simulink model "ModelosTFG"  (R2024b)
settings: Solver=VariableStepAuto  StartTime=0.0  StopTime=75000  RelTol=1e-3
undefined symbols (not defined in the file): Gb, Ib, n, p1, p2, p3, Vi
libraries: slpidlib x2
settings Model: Creator=HP  LastModifiedBy=HP

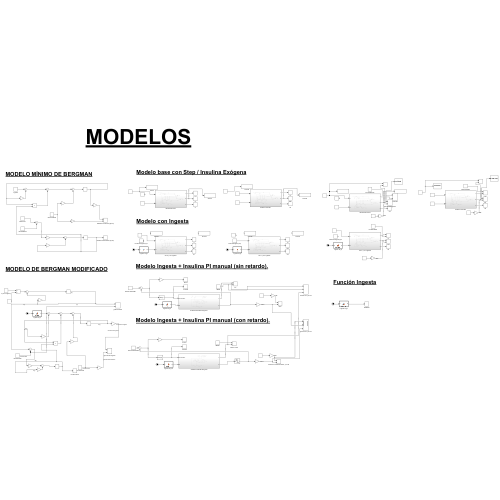
[thumbnail: Simulink's stored preview of the top-level diagram]
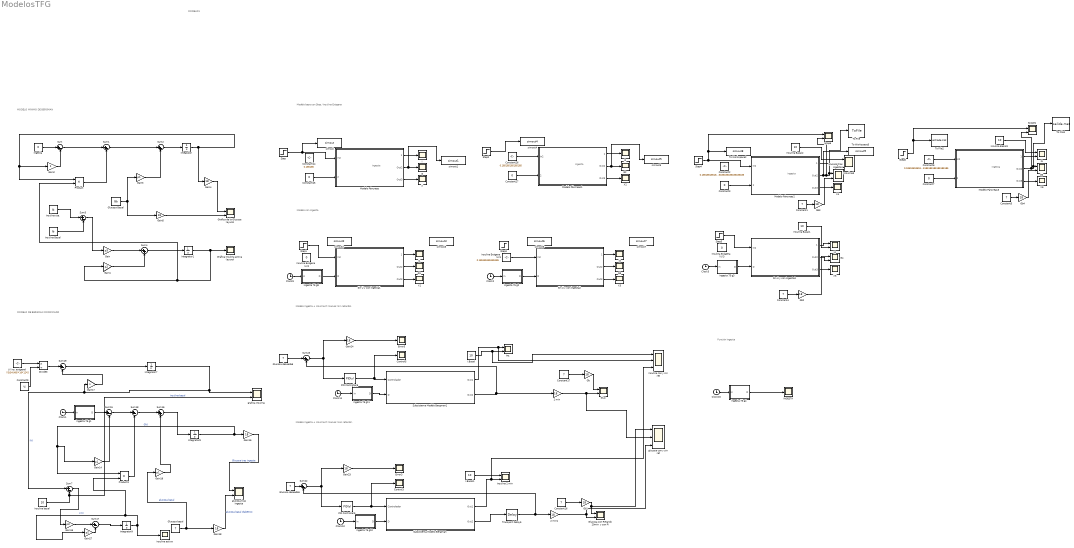
== system ModelosTFG ==
  note: ingesta
  note: Modelo Ingesta + Insulina PI manual (sin retardo).
  note: MODELOS
  note: Función Ingesta
  note: Modelo con Ingesta
  note: ingesta
  note: Modelo base con Step / Insulina Exógena
  note: Modelo Ingesta + Insulina PI manual (con retardo).
  note: MODELO MÍNIMO DE BERGMAN
  note: MODELO DE BERGMAN MODIFICADO
  note: ingesta
  note: ingesta
  2 min : Gain  Gain=18
  2 min1 : Gain  Gain=18
  Clock{1..3,9..11,15} (7 alike) : Clock
  Constant{1,4..5,16..17} (5 alike) : Constant  Value=7
  Constant14 : Constant  Value=0.185185
  Constant{3,7,15,27} (4 alike) : Constant  Value=0
  Constant2 : Constant  Value=0.185185185185185185185185185185
  Constant26 : Constant  Value=0.185185185185185
  Constant6 : Constant  Value=0.185185185185185185185185185185
  Constant9 : Constant  Value=Vi
  Control3 : Scope
  Control5 : Scope
  Divide3 : Product  Inputs=*/
  Error3 : Scope
  Error5 : Scope
  G{,1..3} (4 alike) : Scope
  G4 : Scope  NumInputPorts=2
  G5 : Scope  NumInputPorts=2
  Gain : Gain  Gain=p3
  Gain1 : Gain  Gain=p2
  Gain14 : Gain  Gain=p1
  Gain15 : Gain  Gain=p3
  Gain{4..5,16,18,23..24} (6 alike) : Gain  Gain=18
  Gain17 : Gain  Gain=n
  Gain19 : Gain  Gain=p1
  Gain2 : Gain
  Gain27 : Gain  Gain=p2
  Gain3 : Gain  Gain=p1
  Gb{,1..4} (5 alike) : Gain  Gain=18
  Gluc : Scope  NumInputPorts=2
  Glucosa Basal : Constant  Value=Gb
  Glucosa basal : Constant  Value=7
  Glucosa con Retardo 20min  y con PI : Scope  NumInputPorts=2
  Glucosa deseada5 : Constant  Value=7
  Glucosa deseada6 : Constant  Value=7
  Gráfica Insulina activa (ayuno) : Scope
  Gráfica de la Glucosa (ayuno) : Scope  NumInputPorts=2
  I{,1..3} (4 alike) : Scope
  I.Basal : Constant  Value=10
  I.Basal1 : Constant  Value=10
  I4 : Scope  NumInputPorts=2
  I5 : Scope  NumInputPorts=2
  INGESTA : Scope
  Ingesta : Constant  Value=0
  Ingesta 75 g1 : MATLAB Function  TreatAsAtomicUnit=on
  Ingesta 75 g10 : MATLAB Function  TreatAsAtomicUnit=on
  Ingesta 75 g11 : MATLAB Function  TreatAsAtomicUnit=on
  Ingesta 75 g2 : MATLAB Function  TreatAsAtomicUnit=on
  Ingesta 75 g3 : MATLAB Function  TreatAsAtomicUnit=on
  Ingesta 75 g4 : MATLAB Function  TreatAsAtomicUnit=on
  Ingesta 75 g9 : MATLAB Function  TreatAsAtomicUnit=on
  Ins. : Scope  NumInputPorts=2
  Insulina 2 min : Scope  NumInputPorts=2
  Insulina Basal : Constant  Value=Ib
  Insulina Basal1 : Constant  Value=10
  Insulina Basal2 : Constant  Value=10
  Insulina Basal3 : Constant  Value=10
  Insulina Exógena (U)1 : Constant  Value=0.185185185185185
  Insulina Exógena (U)2 : Constant  Value=0
  Insulina Exógena (U)3 : Constant  Value=0
  Insulina basal : Constant  Value=10
  Insulina cte. : Constant  Value=Ib
  Integrator : Integrator  InitialCondition=4.5
  Integrator1 : Integrator
  Integrator7 : Integrator  InitialCondition=10
  Integrator8 : Integrator  InitialCondition=7
  Integrator9 : Integrator
  Modelo Páncreas : Subsystem
  Modelo Páncreas1 : Subsystem
  Modelo Páncreas2 : Subsystem
  Modelo Páncreas3 : Subsystem
  PID Controller5 : slpidlib/PID Controller  Controller=PID  Form=Parallel  TimeDomain=Continuous-time  UseExternalTs=off  SampleTime=-1  IntegratorMethod=Forward Euler  FilterMethod=Forward Euler  ControllerParametersSource=internal  P=-0.3195  I=-0.3195/2998.95  UseKiTs=off  D=0  UseExternalDerivativeSource=off  N=10  UseFilter=on  TunerSelectOption=Transfer Function Based (PID Tuner App)  InitialConditionSource=internal  InitialConditionForIntegrator=0  InitialConditionForFilter=0  DifferentiatorICPrevScaledInput=0  ExternalReset=none  TrackingMode=off  Kt=1  LimitOutput=off  SatLimitsSource=internal  UpperSaturationLimit=inf  LowerSaturationLimit=-inf  LinearizeAsGain=on  AntiWindupMode=none  Kb=1  LimitIntegrator=off  UpperIntegratorSaturationLimit=inf  LowerIntegratorSaturationLimit=-inf  POutMin=[]  POutMax=[]  IOutMin=[]  IOutMax=[]  DOutMin=[]  DOutMax=[]  NOutMin=[]  NOutMax=[]  SumOutMin=[]  SumOutMax=[]  SaturationOutMin=[]  SaturationOutMax=[]  PParamMin=[]  PParamMax=[]  IParamMin=[]  IParamMax=[]  DParamMin=[]  DParamMax=[]  NParamMin=[]  NParamMax=[]  KbParamMin=[]  KbParamMax=[]  KtParamMin=[]  KtParamMax=[]  KbOutMin=[]  KbOutMax=[]  KtOutMin=[]  KtOutMax=[]  IntegratorOutMin=[]  IntegratorOutMax=[]  FilterOutMin=[]  FilterOutMax=[]  SumI1OutMin=[]  SumI1OutMax=[]  SumI2OutMin=[]  SumI2OutMax=[]  SumI3OutMin=[]  SumI3OutMax=[]  SumI4OutMin=[]  SumI4OutMax=[]  SumDOutMin=[]  SumDOutMax=[]  DifferentiatorOutMin=[]  DifferentiatorOutMax=[]  FilterDiffOutCoefMin=[]  FilterDiffOutCoefMax=[]  ReciprocalOutMin=[]  ReciprocalOutMax=[]  SumDenOutMin=[]  SumDenOutMax=[]  SumNumOutMin=[]  SumNumOutMax=[]  DivideOutMin=[]  DivideOutMax=[]  UdiffTsProdOutMin=[]  UdiffTsProdOutMax=[]  NTsProdOutMin=[]  NTsProdOutMax=[]  UintegralTsProdOutMin=[]  UintegralTsProdOutMax=[]  UngainTsProdOutMin=[]  UngainTsProdOutMax=[]  ClampingZeroOutDataTypeStr=Inherit: Inherit via back propagation  ClampingZeroOutMin=[]  ClampingZeroOutMax=[]  FilterDenConstantOutDataTypeStr=Inherit: Inherit via back propagation  FilterDenConstantOutMin=[]  FilterDenConstantOutMax=[]  PCopyOutDataTypeStr=Inherit: Inherit via back propagation  PCopyOutMin=[]  PCopyOutMax=[]  NCopyOutDataTypeStr=Inherit: Inherit via back propagation  NCopyOutMin=[]  NCopyOutMax=[]  IntegratorContinuousStateAttributes=''  IntegratorStateMustResolveToSignalObject=off  IntegratorRTWStateStorageClass=Auto  FilterContinuousStateAttributes=''  FilterStateMustResolveToSignalObject=off  FilterRTWStateStorageClass=Auto  ParallelPVariant=InternalParameters  IdealPVariant=Disabled  IVariant=InternalParameters  DVariant=InternalParameters  IntegratorVariant=Continuous  SatVariant=Disabled  AWVariant=Passthrough  PCopyVariant=Disabled  TRVariant=Disabled  FdbkBlocksVariant=Forward  IdealPFdbkVariant=Disabled  SatFdbkVariant=Disabled  DerivativeFilterVariant=ContFilter  NVariant=InternalParameters  NCopyVariant=Disabled  FilterICVariant=InternalICsFilter  IntegratorICVariant=InternalICs  ExternalResetVariant=Disabled  TRSumVariant=Passthrough  SumFdbkVariant=Disabled  SumVariant=Sum_PID  TsampFilterVariant=InternalTs  TsampNgainVariant=Passthrough  TsampIntegralVariant=Disabled_SignalSpec  ExternalSaturationOutDataTypeStr=Inherit: Same as second input  DerivativeSourceVariant=ErrorSignal  PreIntVariant=InternalPreInt
  PID Controller6 : slpidlib/PID Controller  Controller=PID  Form=Parallel  TimeDomain=Continuous-time  UseExternalTs=off  SampleTime=-1  IntegratorMethod=Forward Euler  FilterMethod=Forward Euler  ControllerParametersSource=internal  P=-0.3195  I=-0.3195/2998.95  UseKiTs=off  D=0  UseExternalDerivativeSource=off  N=10  UseFilter=on  TunerSelectOption=Transfer Function Based (PID Tuner App)  InitialConditionSource=internal  InitialConditionForIntegrator=0  InitialConditionForFilter=0  DifferentiatorICPrevScaledInput=0  ExternalReset=none  TrackingMode=off  Kt=1  LimitOutput=off  SatLimitsSource=internal  UpperSaturationLimit=inf  LowerSaturationLimit=-inf  LinearizeAsGain=on  AntiWindupMode=none  Kb=1  LimitIntegrator=off  UpperIntegratorSaturationLimit=inf  LowerIntegratorSaturationLimit=-inf  POutMin=[]  POutMax=[]  IOutMin=[]  IOutMax=[]  DOutMin=[]  DOutMax=[]  NOutMin=[]  NOutMax=[]  SumOutMin=[]  SumOutMax=[]  SaturationOutMin=[]  SaturationOutMax=[]  PParamMin=[]  PParamMax=[]  IParamMin=[]  IParamMax=[]  DParamMin=[]  DParamMax=[]  NParamMin=[]  NParamMax=[]  KbParamMin=[]  KbParamMax=[]  KtParamMin=[]  KtParamMax=[]  KbOutMin=[]  KbOutMax=[]  KtOutMin=[]  KtOutMax=[]  IntegratorOutMin=[]  IntegratorOutMax=[]  FilterOutMin=[]  FilterOutMax=[]  SumI1OutMin=[]  SumI1OutMax=[]  SumI2OutMin=[]  SumI2OutMax=[]  SumI3OutMin=[]  SumI3OutMax=[]  SumI4OutMin=[]  SumI4OutMax=[]  SumDOutMin=[]  SumDOutMax=[]  DifferentiatorOutMin=[]  DifferentiatorOutMax=[]  FilterDiffOutCoefMin=[]  FilterDiffOutCoefMax=[]  ReciprocalOutMin=[]  ReciprocalOutMax=[]  SumDenOutMin=[]  SumDenOutMax=[]  SumNumOutMin=[]  SumNumOutMax=[]  DivideOutMin=[]  DivideOutMax=[]  UdiffTsProdOutMin=[]  UdiffTsProdOutMax=[]  NTsProdOutMin=[]  NTsProdOutMax=[]  UintegralTsProdOutMin=[]  UintegralTsProdOutMax=[]  UngainTsProdOutMin=[]  UngainTsProdOutMax=[]  ClampingZeroOutDataTypeStr=Inherit: Inherit via back propagation  ClampingZeroOutMin=[]  ClampingZeroOutMax=[]  FilterDenConstantOutDataTypeStr=Inherit: Inherit via back propagation  FilterDenConstantOutMin=[]  FilterDenConstantOutMax=[]  PCopyOutDataTypeStr=Inherit: Inherit via back propagation  PCopyOutMin=[]  PCopyOutMax=[]  NCopyOutDataTypeStr=Inherit: Inherit via back propagation  NCopyOutMin=[]  NCopyOutMax=[]  IntegratorContinuousStateAttributes=''  IntegratorStateMustResolveToSignalObject=off  IntegratorRTWStateStorageClass=Auto  FilterContinuousStateAttributes=''  FilterStateMustResolveToSignalObject=off  FilterRTWStateStorageClass=Auto  ParallelPVariant=InternalParameters  IdealPVariant=Disabled  IVariant=InternalParameters  DVariant=InternalParameters  IntegratorVariant=Continuous  SatVariant=Disabled  AWVariant=Passthrough  PCopyVariant=Disabled  TRVariant=Disabled  FdbkBlocksVariant=Forward  IdealPFdbkVariant=Disabled  SatFdbkVariant=Disabled  DerivativeFilterVariant=ContFilter  NVariant=InternalParameters  NCopyVariant=Disabled  FilterICVariant=InternalICsFilter  IntegratorICVariant=InternalICs  ExternalResetVariant=Disabled  TRSumVariant=Passthrough  SumFdbkVariant=Disabled  SumVariant=Sum_PID  TsampFilterVariant=InternalTs  TsampNgainVariant=Passthrough  TsampIntegralVariant=Disabled_SignalSpec  ExternalSaturationOutDataTypeStr=Inherit: Same as second input  DerivativeSourceVariant=ErrorSignal  PreIntVariant=InternalPreInt
  Product : Product
  Product3 : Product
  Scope : Scope  NumInputPorts=2
  Scope1 : Scope  NumInputPorts=2
  Sin U y con Ingesta1 : Subsystem
  Sin U y con Ingesta2 : Subsystem
  Sin U y con Ingesta3 : Subsystem
  Step{,1..3,5} (5 alike) : Step  Time=100  Before=0.185185  After=1.185185  SampleTime=0
  Step4 : Step  Time=2000  Before=0.185185185185  After=1.185185  SampleTime=0
  Step6 : Step  Time=2000  Before=0.185185  After=1.185185  SampleTime=0
  Subsistema Modelo Bergman : Subsystem
  Subsistema Modelo Bergman1 : Subsystem
  Sum{,1,3,7,15,17..19,22..23} (10 alike) : Sum  Inputs=|+-
  Sum16 : Sum  Inputs=|++
  Sum2 : Sum  Inputs=|++
  Sum4 : Sum  Inputs=|++
  To File : ToFile  SampleTime=100
  To File1 : ToFile  Filename=salida.mat  MatrixName=glucosa
  To File2 : ToFile  Filename=entrada.mat  MatrixName=Insulina
  To Workspace2 : ToWorkspace  VariableName=simout8  SaveFormat=Timeseries  SampleTime=-1
  To Workspace3 : ToWorkspace  VariableName=simout9  SaveFormat=Timeseries  SampleTime=-1
  Transport Delay5 : TransportDelay  DelayTime=900  InitialOutput=7
  "U (ins. exógena) " : Constant  Value=((5/54)/60)*10*12*5
  X{,1..6} (7 alike) : Scope
  glucosa con y sin ret : Scope  NumInputPorts=3
  glucosa tras ingesta : Scope  NumInputPorts=2
  glucosa tras ingesta1 : Scope  NumInputPorts=2
  grafica insulina : Scope  NumInputPorts=2
  insulina activa : Scope
  insulina con y sin ret : Scope  NumInputPorts=3
  insulina3 : Scope  NumInputPorts=2
  simout : ToWorkspace  VariableName=simout  SaveFormat=Timeseries  SampleTime=-1
  simout1 : ToWorkspace  VariableName=simout1  SaveFormat=Timeseries  SampleTime=-1
  simout2 : ToWorkspace  VariableName=simout2  SaveFormat=Timeseries  SampleTime=-1
  simout3 : ToWorkspace  VariableName=simout3  SaveFormat=Timeseries  SampleTime=-1
  simout4 : ToWorkspace  VariableName=simout4  SaveFormat=Timeseries  SampleTime=-1
  simout5 : ToWorkspace  VariableName=simout5  SaveFormat=Timeseries  SampleTime=-1
  simout6 : ToWorkspace  VariableName=simout6  SaveFormat=Timeseries  SampleTime=-1
  simout7 : ToWorkspace  VariableName=simout7  SaveFormat=Timeseries  SampleTime=-1
  wires:
  Clock10/1 -> Ingesta 75 g10/1(in)
  Modelo Páncreas1/2(Out2) -> simout5/1, G2/1
  Modelo Páncreas/2(Out2) -> simout1/1, G/1
  Step2/1 -> simout4/1
  PID Controller6/1 -> Control5/1, Subsistema Modelo Bergman1/1(Controlador)
  Modelo Páncreas/1(1) -> I/1
  I.Basal1/1 -> Insulina 2 min/1
  Constant16/1 -> Gb1/1
  I.Basal/1 -> insulina con y sin ret/1, Ins./2
  Constant17/1 -> Gb/1
  Sum23/1 -> PID Controller6/1, Gain24/1
  Step/1 -> simout/1, Modelo Páncreas/1(In2)
  Glucosa deseada5/1 -> Sum22/1
  Ingesta 75 g11/1(D) -> Subsistema Modelo Bergman1/2(D)
  2 min/1 -> glucosa con y sin ret/2, Gluc/2
  Step1/1 -> Sin U y con Ingesta1/1(In2)
  Clock11/1 -> Ingesta 75 g11/1(in)
  2 min1/1 -> glucosa con y sin ret/3, Glucosa con Retardo 20min  y con PI/2
  Clock9/1 -> Ingesta 75 g9/1(in)
  Constant26/1 -> Modelo Páncreas1/1(In2)
  Ingesta 75 g9/1(D) -> Sin U y con Ingesta1/2(D)
  Gb1/1 -> Glucosa con Retardo 20min  y con PI/1, glucosa con y sin ret/1
  Sin U y con Ingesta1/1(1) -> I1/1
  Subsistema Modelo Bergman1/1(Out1) -> insulina con y sin ret/2, Ins./1
  Constant27/1 -> Modelo Páncreas1/2(2)
  Sin U y con Ingesta1/3(Out3) -> X1/1
  Sum22/1 -> PID Controller5/1, Gain23/1
  Glucosa deseada6/1 -> Sum23/1
  Gb/1 -> Gluc/1
  Subsistema Modelo Bergman1/2(Out2) -> Sum23/2, 2 min/1
  Modelo Páncreas1/1(1) -> I2/1
  Clock15/1 -> Ingesta 75 g4/1(in)
  PID Controller5/1 -> Control3/1, Subsistema Modelo Bergman/1(Controlador)
  Subsistema Modelo Bergman/2(Out2) -> Transport Delay5/1
  Modelo Páncreas/3(Out3) -> X/1
  Ingesta 75 g4/1(D) -> INGESTA/1
  Subsistema Modelo Bergman/1(Out1) -> insulina con y sin ret/3, Insulina 2 min/2
  Gain23/1 -> Error3/1
  Transport Delay5/1 -> Sum22/2, 2 min1/1
  Ingesta 75 g10/1(D) -> Subsistema Modelo Bergman/2(D)
  Modelo Páncreas1/3(Out3) -> X2/1
  Gain24/1 -> Error5/1
  Constant15/1 -> Modelo Páncreas/2(2)
  Sin U y con Ingesta1/2(Out2) -> G1/1
  Glucosa Basal/1 -> Gain3/1, Gain5/1
  Sum/1 -> Sum1/1
  Insulina cte./1 -> Sum3/1
  Sum4/1 -> Integrator1/1
  Ingesta/1 -> Sum/1
  Gain4/1 -> Gráfica de la Glucosa (ayuno)/1
  Sum2/1 -> Integrator/1
  Gain3/1 -> Sum2/2
  Gain1/1 -> Sum4/2
  Integrator/1 -> Gain4/1, Product/1, Gain2/1
  Sum3/1 -> Gain/1
  Gain/1 -> Sum4/1
  Integrator1/1 -> Product/2, Gain1/1, Gráfica Insulina activa (ayuno)/1
  Insulina Basal/1 -> Sum3/2
  Product/1 -> Sum1/2
  Sum1/1 -> Sum2/1
  Gain2/1 -> Sum/2
  Sum15/1 -> Sum18/1
  Integrator9/1 -> insulina activa/1, Product3/2, Gain27/1  "X(t)"
  Divide3/1 -> Sum19/1
  Gain14/1 -> Sum15/2
  Insulina basal/1 -> grafica insulina/2, Sum7/2  "insulina basal"
  Sum18/1 -> Sum16/1
  Gain27/1 -> Sum17/2
  Gain19/1 -> Sum16/2
  Glucosa basal/1 -> Gain19/1, Gain18/1  "glucosa basal"
  Integrator7/1 -> Sum7/1, Gain17/1, grafica insulina/1  "I(t)"
  Sum16/1 -> Integrator8/1
  Clock1/1 -> Ingesta 75 g1/1(in)
  Ingesta 75 g1/1(D) -> Sum15/1
  Integrator8/1 -> Gain16/1, Product3/1, Gain14/1  "G(t)"
  Gain17/1 -> Sum19/2
  Gain16/1 -> glucosa tras ingesta/1  "Glucosa tras ingesta"
  Product3/1 -> Sum18/2
  Gain18/1 -> glucosa tras ingesta/2  "glucosa basal diabetico"
  Sum17/1 -> Integrator9/1
  Sum19/1 -> Integrator7/1
  Sum7/1 -> Gain15/1
  "U (ins. exógena) "/1 -> Divide3/1
  Constant9/1 -> Divide3/2
  Gain15/1 -> Sum17/1
  Gain5/1 -> Gráfica de la Glucosa (ayuno)/2
  Sin U y con Ingesta2/2(Out2) -> G3/1
  Ingesta 75 g2/1(D) -> Sin U y con Ingesta2/2(D)
  Sin U y con Ingesta2/1(1) -> I3/1
  Sin U y con Ingesta2/3(Out3) -> X3/1
  Clock2/1 -> Ingesta 75 g2/1(in)
  Insulina Exógena (U)1/1 -> Sin U y con Ingesta2/1(In2)
  Insulina Basal2/1 -> insulina3/1
  Modelo Páncreas2/1(1) -> insulina3/2
  Gb3/1 -> glucosa tras ingesta1/2
  Modelo Páncreas2/2(Out2) -> To Workspace3/1, Scope/2, glucosa tras ingesta1/1, To File/1
  Step5/1 -> Sin U y con Ingesta3/1(In2)
  Modelo Páncreas3/2(Out2) -> Scope1/2, G5/1, To File1/1
  Modelo Páncreas3/3(Out3) -> X6/1
  Sin U y con Ingesta3/1(1) -> I4/1
  Constant3/1 -> Modelo Páncreas2/2(2)
  Modelo Páncreas3/1(1) -> I5/2
  Constant6/1 -> Modelo Páncreas3/1(In2)
  Step4/1 -> To Workspace2/1, Scope/1, Modelo Páncreas2/1(In2)
  Insulina Basal3/1 -> I5/1
  Sin U y con Ingesta3/2(Out2) -> G4/2
  Insulina Basal1/1 -> I4/2
  Gb4/1 -> G5/2
  Gb2/1 -> G4/1
  Ingesta 75 g3/1(D) -> Sin U y con Ingesta3/2(D)
  Constant5/1 -> Gb4/1
  Clock3/1 -> Ingesta 75 g3/1(in)
  Sin U y con Ingesta3/3(Out3) -> X5/1
  Step6/1 -> Scope1/1, To File2/1
  Constant7/1 -> Modelo Páncreas3/2(2)
  Constant1/1 -> Gb3/1
  Constant4/1 -> Gb2/1
  Modelo Páncreas2/3(Out3) -> X4/1

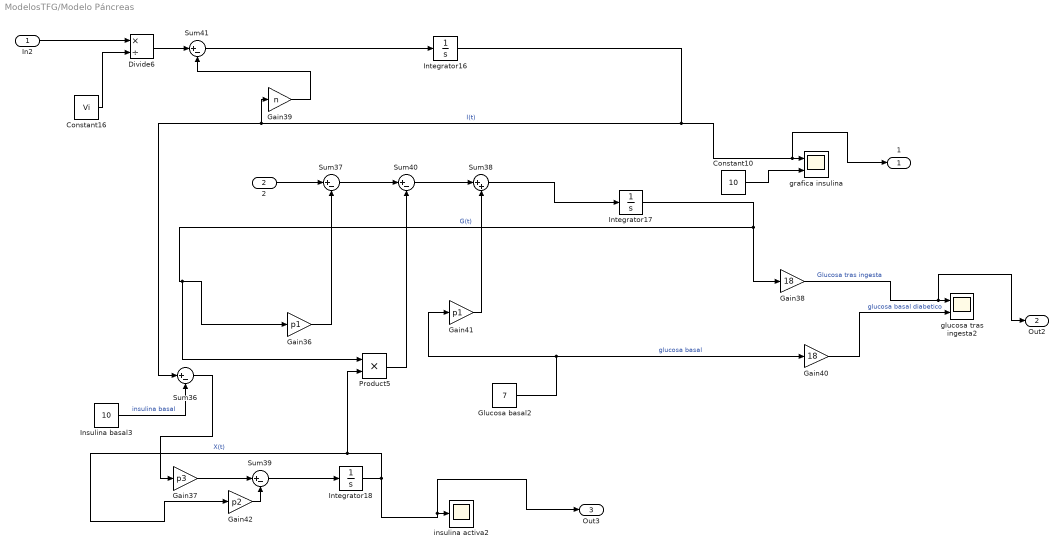
== system ModelosTFG/Modelo Páncreas ==
  In2 : Inport
  2 : Inport  Port=2
  Constant10 : Constant  Value=10
  Constant16 : Constant  Value=Vi
  Divide6 : Product  Inputs=*/
  Gain36 : Gain  Gain=p1
  Gain37 : Gain  Gain=p3
  Gain38 : Gain  Gain=18
  Gain39 : Gain  Gain=n
  Gain40 : Gain  Gain=18
  Gain41 : Gain  Gain=p1
  Gain42 : Gain  Gain=p2
  Glucosa basal2 : Constant  Value=7
  Insulina basal3 : Constant  Value=10
  Integrator16 : Integrator  InitialCondition=10
  Integrator17 : Integrator  InitialCondition=7
  Integrator18 : Integrator
  Product5 : Product
  Sum{36..37,39..41} (5 alike) : Sum  Inputs=|+-
  Sum38 : Sum  Inputs=|++
  glucosa tras ingesta2 : Scope  NumInputPorts=2
  grafica insulina : Scope  NumInputPorts=2
  insulina activa2 : Scope
  1 : Outport
  Out2 : Outport  Port=2
  Out3 : Outport  Port=3
  wires:
  Integrator18/1 -> Out3/1, insulina activa2/1, Product5/2, Gain42/1  "X(t)"
  Integrator17/1 -> Gain38/1, Product5/1, Gain36/1  "G(t)"
  Gain39/1 -> Sum41/2
  Glucosa basal2/1 -> Gain41/1, Gain40/1  "glucosa basal"
  Integrator16/1 -> Sum36/1, Gain39/1, 1/1, grafica insulina/1  "I(t)"
  Constant10/1 -> grafica insulina/2
  Gain42/1 -> Sum39/2
  2/1 -> Sum37/1
  Sum37/1 -> Sum40/1
  Sum39/1 -> Integrator18/1
  Gain40/1 -> glucosa tras ingesta2/2  "glucosa basal diabetico"
  Sum40/1 -> Sum38/1
  In2/1 -> Divide6/1
  Gain36/1 -> Sum37/2
  Gain38/1 -> Out2/1, glucosa tras ingesta2/1  "Glucosa tras ingesta"
  Sum36/1 -> Gain37/1
  Gain41/1 -> Sum38/2
  Gain37/1 -> Sum39/1
  Sum41/1 -> Integrator16/1
  Sum38/1 -> Integrator17/1
  Insulina basal3/1 -> Sum36/2  "insulina basal"
  Divide6/1 -> Sum41/1
  Constant16/1 -> Divide6/2
  Product5/1 -> Sum40/2

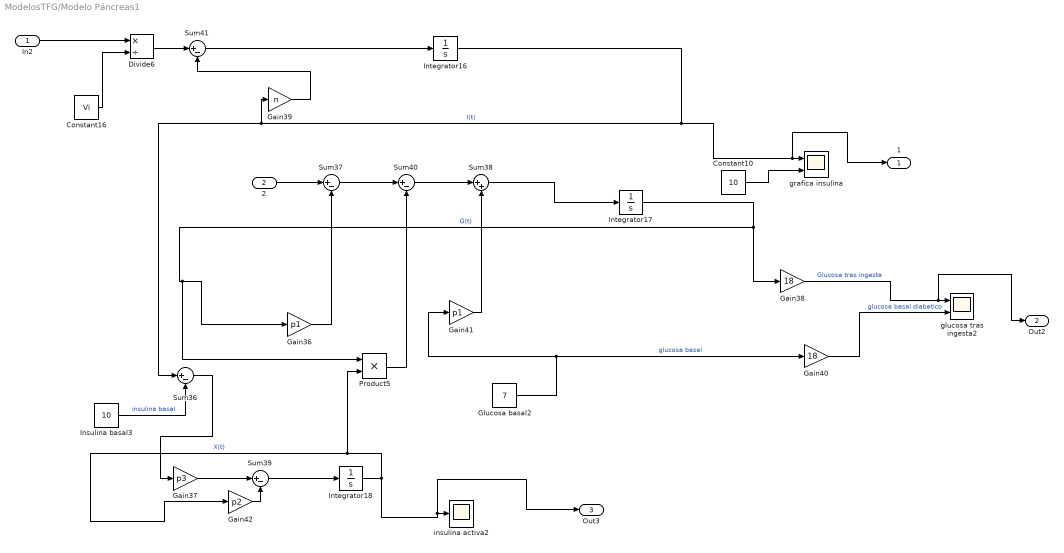
== system ModelosTFG/Modelo Páncreas1 ==
  In2 : Inport
  2 : Inport  Port=2
  Constant10 : Constant  Value=10
  Constant16 : Constant  Value=Vi
  Divide6 : Product  Inputs=*/
  Gain36 : Gain  Gain=p1
  Gain37 : Gain  Gain=p3
  Gain38 : Gain  Gain=18
  Gain39 : Gain  Gain=n
  Gain40 : Gain  Gain=18
  Gain41 : Gain  Gain=p1
  Gain42 : Gain  Gain=p2
  Glucosa basal2 : Constant  Value=7
  Insulina basal3 : Constant  Value=10
  Integrator16 : Integrator  InitialCondition=10
  Integrator17 : Integrator  InitialCondition=7
  Integrator18 : Integrator
  Product5 : Product
  Sum{36..37,39..41} (5 alike) : Sum  Inputs=|+-
  Sum38 : Sum  Inputs=|++
  glucosa tras ingesta2 : Scope  NumInputPorts=2
  grafica insulina : Scope  NumInputPorts=2
  insulina activa2 : Scope
  1 : Outport
  Out2 : Outport  Port=2
  Out3 : Outport  Port=3
  wires:
  Integrator18/1 -> Out3/1, insulina activa2/1, Product5/2, Gain42/1  "X(t)"
  Integrator17/1 -> Gain38/1, Product5/1, Gain36/1  "G(t)"
  Gain39/1 -> Sum41/2
  Glucosa basal2/1 -> Gain41/1, Gain40/1  "glucosa basal"
  Integrator16/1 -> Sum36/1, Gain39/1, 1/1, grafica insulina/1  "I(t)"
  Constant10/1 -> grafica insulina/2
  Gain42/1 -> Sum39/2
  2/1 -> Sum37/1
  Sum37/1 -> Sum40/1
  Sum39/1 -> Integrator18/1
  Gain40/1 -> glucosa tras ingesta2/2  "glucosa basal diabetico"
  Sum40/1 -> Sum38/1
  In2/1 -> Divide6/1
  Gain36/1 -> Sum37/2
  Gain38/1 -> Out2/1, glucosa tras ingesta2/1  "Glucosa tras ingesta"
  Sum36/1 -> Gain37/1
  Gain41/1 -> Sum38/2
  Gain37/1 -> Sum39/1
  Sum41/1 -> Integrator16/1
  Sum38/1 -> Integrator17/1
  Insulina basal3/1 -> Sum36/2  "insulina basal"
  Divide6/1 -> Sum41/1
  Constant16/1 -> Divide6/2
  Product5/1 -> Sum40/2

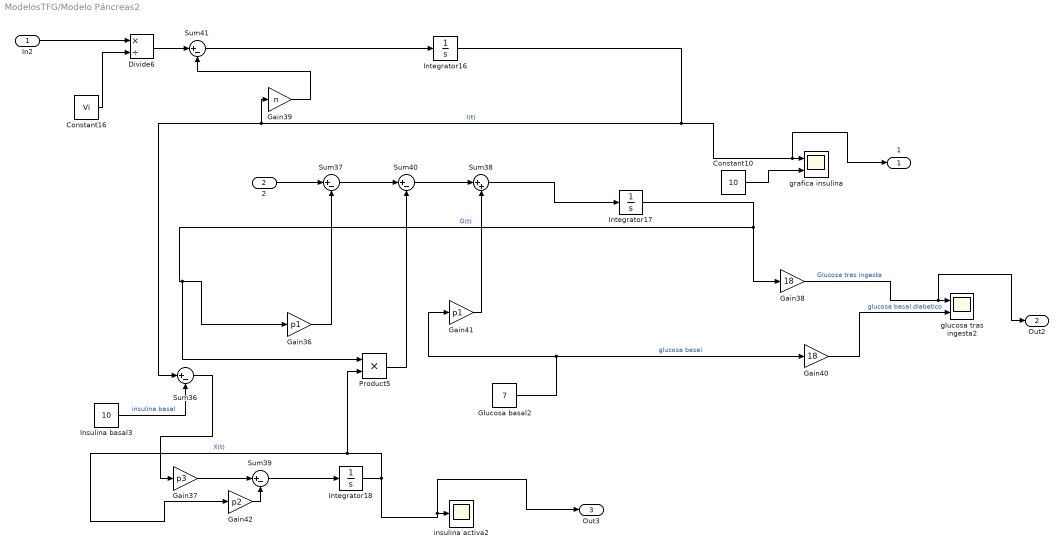
== system ModelosTFG/Modelo Páncreas2 ==
  In2 : Inport
  2 : Inport  Port=2
  Constant10 : Constant  Value=10
  Constant16 : Constant  Value=Vi
  Divide6 : Product  Inputs=*/
  Gain36 : Gain  Gain=p1
  Gain37 : Gain  Gain=p3
  Gain38 : Gain  Gain=18
  Gain39 : Gain  Gain=n
  Gain40 : Gain  Gain=18
  Gain41 : Gain  Gain=p1
  Gain42 : Gain  Gain=p2
  Glucosa basal2 : Constant  Value=7
  Insulina basal3 : Constant  Value=10
  Integrator16 : Integrator  InitialCondition=10
  Integrator17 : Integrator  InitialCondition=7
  Integrator18 : Integrator
  Product5 : Product
  Sum{36..37,39..41} (5 alike) : Sum  Inputs=|+-
  Sum38 : Sum  Inputs=|++
  glucosa tras ingesta2 : Scope  NumInputPorts=2
  grafica insulina : Scope  NumInputPorts=2
  insulina activa2 : Scope
  1 : Outport
  Out2 : Outport  Port=2
  Out3 : Outport  Port=3
  wires:
  Integrator18/1 -> Out3/1, insulina activa2/1, Product5/2, Gain42/1  "X(t)"
  Integrator17/1 -> Gain38/1, Product5/1, Gain36/1  "G(t)"
  Gain39/1 -> Sum41/2
  Glucosa basal2/1 -> Gain41/1, Gain40/1  "glucosa basal"
  Integrator16/1 -> Sum36/1, Gain39/1, 1/1, grafica insulina/1  "I(t)"
  Constant10/1 -> grafica insulina/2
  Gain42/1 -> Sum39/2
  2/1 -> Sum37/1
  Sum37/1 -> Sum40/1
  Sum39/1 -> Integrator18/1
  Gain40/1 -> glucosa tras ingesta2/2  "glucosa basal diabetico"
  Sum40/1 -> Sum38/1
  In2/1 -> Divide6/1
  Gain36/1 -> Sum37/2
  Gain38/1 -> Out2/1, glucosa tras ingesta2/1  "Glucosa tras ingesta"
  Sum36/1 -> Gain37/1
  Gain41/1 -> Sum38/2
  Gain37/1 -> Sum39/1
  Sum41/1 -> Integrator16/1
  Sum38/1 -> Integrator17/1
  Insulina basal3/1 -> Sum36/2  "insulina basal"
  Divide6/1 -> Sum41/1
  Constant16/1 -> Divide6/2
  Product5/1 -> Sum40/2

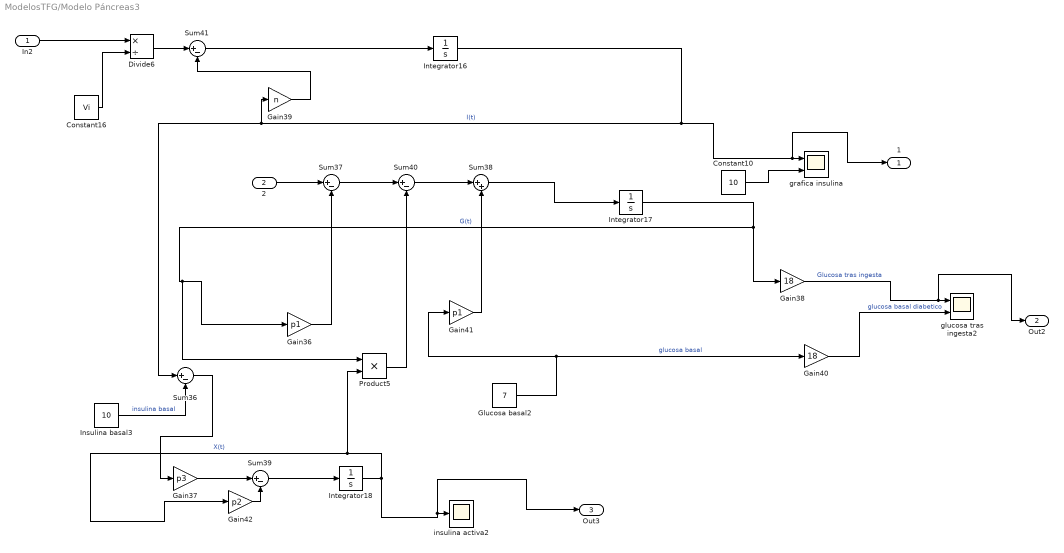
== system ModelosTFG/Modelo Páncreas3 ==
  In2 : Inport
  2 : Inport  Port=2
  Constant10 : Constant  Value=10
  Constant16 : Constant  Value=Vi
  Divide6 : Product  Inputs=*/
  Gain36 : Gain  Gain=p1
  Gain37 : Gain  Gain=p3
  Gain38 : Gain  Gain=18
  Gain39 : Gain  Gain=n
  Gain40 : Gain  Gain=18
  Gain41 : Gain  Gain=p1
  Gain42 : Gain  Gain=p2
  Glucosa basal2 : Constant  Value=7
  Insulina basal3 : Constant  Value=10
  Integrator16 : Integrator  InitialCondition=10
  Integrator17 : Integrator  InitialCondition=7
  Integrator18 : Integrator
  Product5 : Product
  Sum{36..37,39..41} (5 alike) : Sum  Inputs=|+-
  Sum38 : Sum  Inputs=|++
  glucosa tras ingesta2 : Scope  NumInputPorts=2
  grafica insulina : Scope  NumInputPorts=2
  insulina activa2 : Scope
  1 : Outport
  Out2 : Outport  Port=2
  Out3 : Outport  Port=3
  wires:
  Integrator18/1 -> Out3/1, insulina activa2/1, Product5/2, Gain42/1  "X(t)"
  Integrator17/1 -> Gain38/1, Product5/1, Gain36/1  "G(t)"
  Gain39/1 -> Sum41/2
  Glucosa basal2/1 -> Gain41/1, Gain40/1  "glucosa basal"
  Integrator16/1 -> Sum36/1, Gain39/1, 1/1, grafica insulina/1  "I(t)"
  Constant10/1 -> grafica insulina/2
  Gain42/1 -> Sum39/2
  2/1 -> Sum37/1
  Sum37/1 -> Sum40/1
  Sum39/1 -> Integrator18/1
  Gain40/1 -> glucosa tras ingesta2/2  "glucosa basal diabetico"
  Sum40/1 -> Sum38/1
  In2/1 -> Divide6/1
  Gain36/1 -> Sum37/2
  Gain38/1 -> Out2/1, glucosa tras ingesta2/1  "Glucosa tras ingesta"
  Sum36/1 -> Gain37/1
  Gain41/1 -> Sum38/2
  Gain37/1 -> Sum39/1
  Sum41/1 -> Integrator16/1
  Sum38/1 -> Integrator17/1
  Insulina basal3/1 -> Sum36/2  "insulina basal"
  Divide6/1 -> Sum41/1
  Constant16/1 -> Divide6/2
  Product5/1 -> Sum40/2

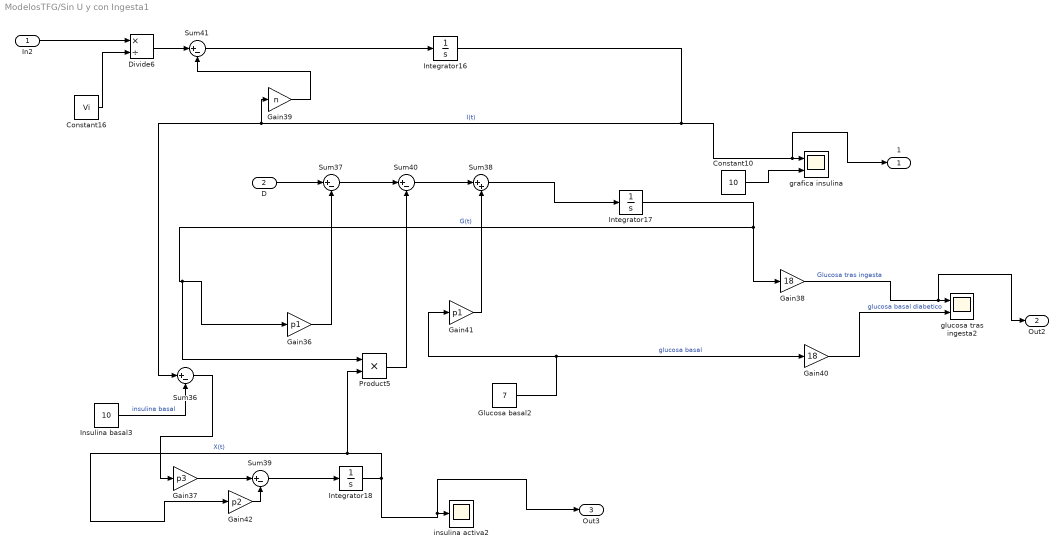
== system ModelosTFG/Sin U y con Ingesta1 ==
  In2 : Inport
  D : Inport  Port=2
  Constant10 : Constant  Value=10
  Constant16 : Constant  Value=Vi
  Divide6 : Product  Inputs=*/
  Gain36 : Gain  Gain=p1
  Gain37 : Gain  Gain=p3
  Gain38 : Gain  Gain=18
  Gain39 : Gain  Gain=n
  Gain40 : Gain  Gain=18
  Gain41 : Gain  Gain=p1
  Gain42 : Gain  Gain=p2
  Glucosa basal2 : Constant  Value=7
  Insulina basal3 : Constant  Value=10
  Integrator16 : Integrator  InitialCondition=10
  Integrator17 : Integrator  InitialCondition=7
  Integrator18 : Integrator
  Product5 : Product
  Sum{36..37,39..41} (5 alike) : Sum  Inputs=|+-
  Sum38 : Sum  Inputs=|++
  glucosa tras ingesta2 : Scope  NumInputPorts=2
  grafica insulina : Scope  NumInputPorts=2
  insulina activa2 : Scope
  1 : Outport
  Out2 : Outport  Port=2
  Out3 : Outport  Port=3
  wires:
  Integrator18/1 -> Out3/1, insulina activa2/1, Product5/2, Gain42/1  "X(t)"
  Integrator17/1 -> Gain38/1, Product5/1, Gain36/1  "G(t)"
  Gain39/1 -> Sum41/2
  Glucosa basal2/1 -> Gain41/1, Gain40/1  "glucosa basal"
  Integrator16/1 -> Sum36/1, Gain39/1, 1/1, grafica insulina/1  "I(t)"
  Constant10/1 -> grafica insulina/2
  Gain42/1 -> Sum39/2
  D/1 -> Sum37/1
  Sum37/1 -> Sum40/1
  Sum39/1 -> Integrator18/1
  Gain40/1 -> glucosa tras ingesta2/2  "glucosa basal diabetico"
  Sum40/1 -> Sum38/1
  In2/1 -> Divide6/1
  Gain36/1 -> Sum37/2
  Gain38/1 -> Out2/1, glucosa tras ingesta2/1  "Glucosa tras ingesta"
  Sum36/1 -> Gain37/1
  Gain41/1 -> Sum38/2
  Gain37/1 -> Sum39/1
  Sum41/1 -> Integrator16/1
  Sum38/1 -> Integrator17/1
  Insulina basal3/1 -> Sum36/2  "insulina basal"
  Divide6/1 -> Sum41/1
  Constant16/1 -> Divide6/2
  Product5/1 -> Sum40/2

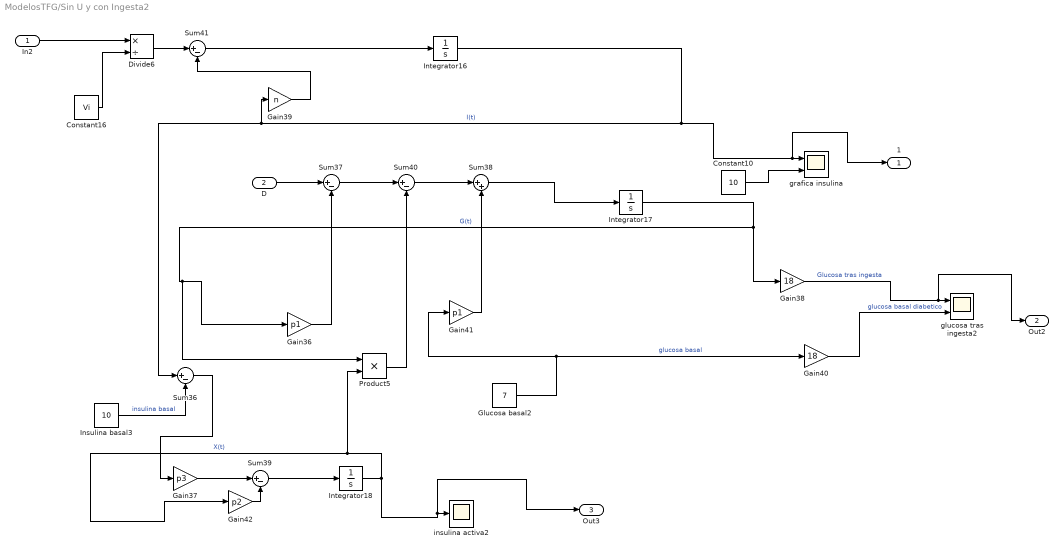
== system ModelosTFG/Sin U y con Ingesta2 ==
  In2 : Inport
  D : Inport  Port=2
  Constant10 : Constant  Value=10
  Constant16 : Constant  Value=Vi
  Divide6 : Product  Inputs=*/
  Gain36 : Gain  Gain=p1
  Gain37 : Gain  Gain=p3
  Gain38 : Gain  Gain=18
  Gain39 : Gain  Gain=n
  Gain40 : Gain  Gain=18
  Gain41 : Gain  Gain=p1
  Gain42 : Gain  Gain=p2
  Glucosa basal2 : Constant  Value=7
  Insulina basal3 : Constant  Value=10
  Integrator16 : Integrator  InitialCondition=10
  Integrator17 : Integrator  InitialCondition=7
  Integrator18 : Integrator
  Product5 : Product
  Sum{36..37,39..41} (5 alike) : Sum  Inputs=|+-
  Sum38 : Sum  Inputs=|++
  glucosa tras ingesta2 : Scope  NumInputPorts=2
  grafica insulina : Scope  NumInputPorts=2
  insulina activa2 : Scope
  1 : Outport
  Out2 : Outport  Port=2
  Out3 : Outport  Port=3
  wires:
  Integrator18/1 -> Out3/1, insulina activa2/1, Product5/2, Gain42/1  "X(t)"
  Integrator17/1 -> Gain38/1, Product5/1, Gain36/1  "G(t)"
  Gain39/1 -> Sum41/2
  Glucosa basal2/1 -> Gain41/1, Gain40/1  "glucosa basal"
  Integrator16/1 -> Sum36/1, Gain39/1, 1/1, grafica insulina/1  "I(t)"
  Constant10/1 -> grafica insulina/2
  Gain42/1 -> Sum39/2
  D/1 -> Sum37/1
  Sum37/1 -> Sum40/1
  Sum39/1 -> Integrator18/1
  Gain40/1 -> glucosa tras ingesta2/2  "glucosa basal diabetico"
  Sum40/1 -> Sum38/1
  In2/1 -> Divide6/1
  Gain36/1 -> Sum37/2
  Gain38/1 -> Out2/1, glucosa tras ingesta2/1  "Glucosa tras ingesta"
  Sum36/1 -> Gain37/1
  Gain41/1 -> Sum38/2
  Gain37/1 -> Sum39/1
  Sum41/1 -> Integrator16/1
  Sum38/1 -> Integrator17/1
  Insulina basal3/1 -> Sum36/2  "insulina basal"
  Divide6/1 -> Sum41/1
  Constant16/1 -> Divide6/2
  Product5/1 -> Sum40/2

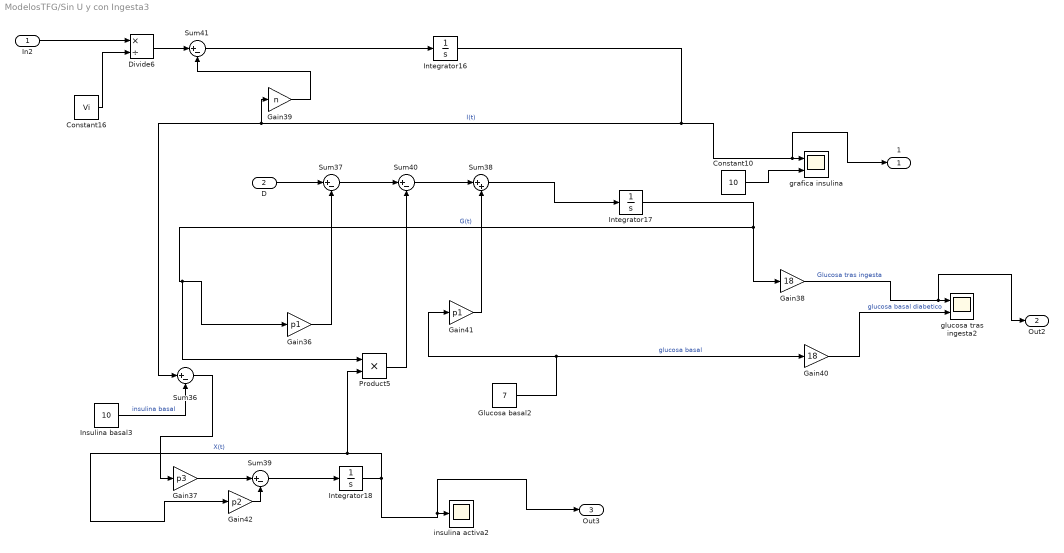
== system ModelosTFG/Sin U y con Ingesta3 ==
  In2 : Inport
  D : Inport  Port=2
  Constant10 : Constant  Value=10
  Constant16 : Constant  Value=Vi
  Divide6 : Product  Inputs=*/
  Gain36 : Gain  Gain=p1
  Gain37 : Gain  Gain=p3
  Gain38 : Gain  Gain=18
  Gain39 : Gain  Gain=n
  Gain40 : Gain  Gain=18
  Gain41 : Gain  Gain=p1
  Gain42 : Gain  Gain=p2
  Glucosa basal2 : Constant  Value=7
  Insulina basal3 : Constant  Value=10
  Integrator16 : Integrator  InitialCondition=10
  Integrator17 : Integrator  InitialCondition=7
  Integrator18 : Integrator
  Product5 : Product
  Sum{36..37,39..41} (5 alike) : Sum  Inputs=|+-
  Sum38 : Sum  Inputs=|++
  glucosa tras ingesta2 : Scope  NumInputPorts=2
  grafica insulina : Scope  NumInputPorts=2
  insulina activa2 : Scope
  1 : Outport
  Out2 : Outport  Port=2
  Out3 : Outport  Port=3
  wires:
  Integrator18/1 -> Out3/1, insulina activa2/1, Product5/2, Gain42/1  "X(t)"
  Integrator17/1 -> Gain38/1, Product5/1, Gain36/1  "G(t)"
  Gain39/1 -> Sum41/2
  Glucosa basal2/1 -> Gain41/1, Gain40/1  "glucosa basal"
  Integrator16/1 -> Sum36/1, Gain39/1, 1/1, grafica insulina/1  "I(t)"
  Constant10/1 -> grafica insulina/2
  Gain42/1 -> Sum39/2
  D/1 -> Sum37/1
  Sum37/1 -> Sum40/1
  Sum39/1 -> Integrator18/1
  Gain40/1 -> glucosa tras ingesta2/2  "glucosa basal diabetico"
  Sum40/1 -> Sum38/1
  In2/1 -> Divide6/1
  Gain36/1 -> Sum37/2
  Gain38/1 -> Out2/1, glucosa tras ingesta2/1  "Glucosa tras ingesta"
  Sum36/1 -> Gain37/1
  Gain41/1 -> Sum38/2
  Gain37/1 -> Sum39/1
  Sum41/1 -> Integrator16/1
  Sum38/1 -> Integrator17/1
  Insulina basal3/1 -> Sum36/2  "insulina basal"
  Divide6/1 -> Sum41/1
  Constant16/1 -> Divide6/2
  Product5/1 -> Sum40/2

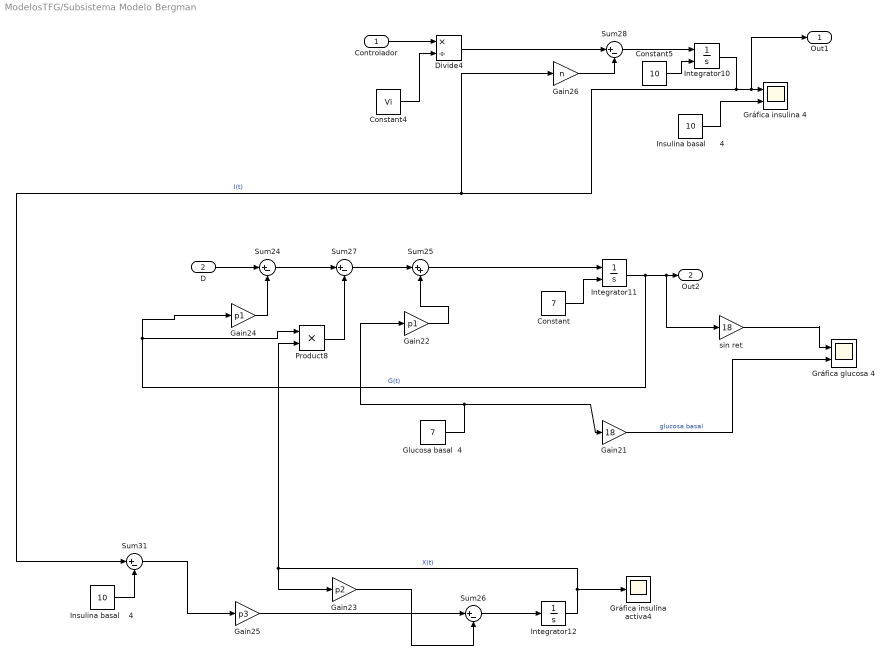
== system ModelosTFG/Subsistema Modelo Bergman ==
  Controlador : Inport
  D : Inport  Port=2
  Constant : Constant  Value=7
  Constant4 : Constant  Value=Vi
  Constant5 : Constant  Value=10
  Divide4 : Product  Inputs=*/
  Gain21 : Gain  Gain=18
  Gain22 : Gain  Gain=p1
  Gain23 : Gain  Gain=p2
  Gain24 : Gain  Gain=p1
  Gain25 : Gain  Gain=p3
  Gain26 : Gain  Gain=n
  Glucosa basal  4 : Constant  Value=7
  Gráfica glucosa 4 : Scope  NumInputPorts=2
  Gráfica insulina 4 : Scope  NumInputPorts=2
  Gráfica insulina activa4 : Scope
  Insulina basal      4 : Constant  Value=10
  Insulina basal    4 : Constant  Value=10
  Integrator10 : Integrator  InitialConditionSource=external
  Integrator11 : Integrator  InitialConditionSource=external  InitialCondition=7
  Integrator12 : Integrator
  Product8 : Product
  Sum{24,26..28,31} (5 alike) : Sum  Inputs=|+-
  Sum25 : Sum  Inputs=|++
  sin ret : Gain  Gain=18
  Out1 : Outport
  Out2 : Outport  Port=2
  wires:
  Gain26/1 -> Sum28/2
  Glucosa basal  4/1 -> Gain22/1, Gain21/1
  D/1 -> Sum24/1
  Gain21/1 -> Gráfica glucosa 4/2  "glucosa basal"
  Integrator11/1 -> sin ret/1, Out2/1, Gain24/1, Product8/1  "G(t)"
  Integrator12/1 -> Product8/2, Gain23/1, Gráfica insulina activa4/1  "X(t)"
  Gain25/1 -> Sum26/1
  Integrator10/1 -> Out1/1, Gráfica insulina 4/1, Sum31/1, Gain26/1  "I(t)"
  Constant5/1 -> Integrator10/2
  Sum31/1 -> Gain25/1
  Sum26/1 -> Integrator12/1
  Gain23/1 -> Sum26/2
  Sum28/1 -> Integrator10/1
  Sum24/1 -> Sum27/1
  Sum25/1 -> Integrator11/1
  Gain24/1 -> Sum24/2
  Insulina basal      4/1 -> Gráfica insulina 4/2
  Sum27/1 -> Sum25/1
  Insulina basal    4/1 -> Sum31/2
  Divide4/1 -> Sum28/1
  Gain22/1 -> Sum25/2
  Product8/1 -> Sum27/2
  Constant4/1 -> Divide4/2
  Constant/1 -> Integrator11/2
  Controlador/1 -> Divide4/1
  sin ret/1 -> Gráfica glucosa 4/1

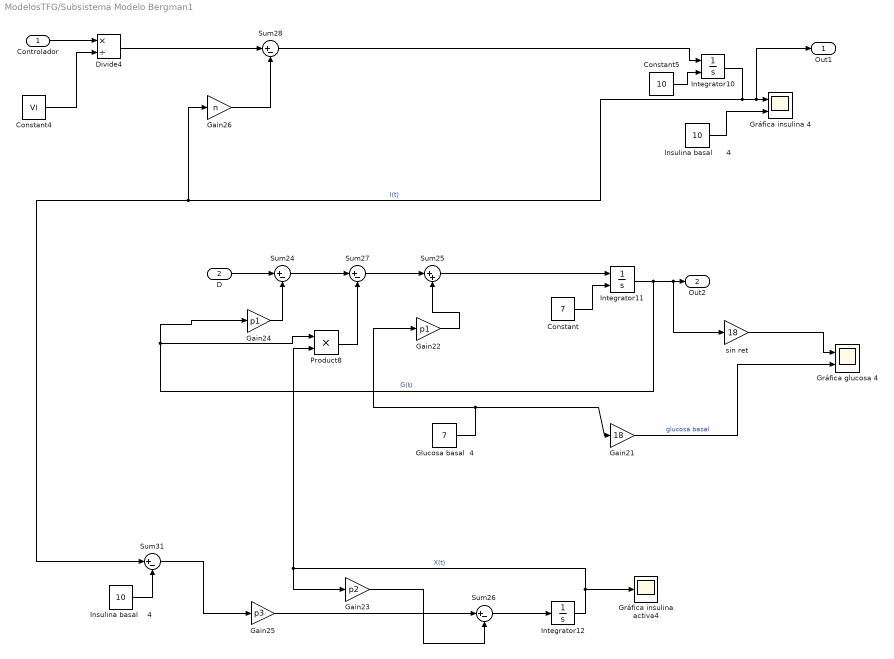
== system ModelosTFG/Subsistema Modelo Bergman1 ==
  Controlador : Inport
  D : Inport  Port=2
  Constant : Constant  Value=7
  Constant4 : Constant  Value=Vi
  Constant5 : Constant  Value=10
  Divide4 : Product  Inputs=*/
  Gain21 : Gain  Gain=18
  Gain22 : Gain  Gain=p1
  Gain23 : Gain  Gain=p2
  Gain24 : Gain  Gain=p1
  Gain25 : Gain  Gain=p3
  Gain26 : Gain  Gain=n
  Glucosa basal  4 : Constant  Value=7
  Gráfica glucosa 4 : Scope  NumInputPorts=2
  Gráfica insulina 4 : Scope  NumInputPorts=2
  Gráfica insulina activa4 : Scope
  Insulina basal      4 : Constant  Value=10
  Insulina basal    4 : Constant  Value=10
  Integrator10 : Integrator  InitialConditionSource=external
  Integrator11 : Integrator  InitialConditionSource=external  InitialCondition=7
  Integrator12 : Integrator
  Product8 : Product
  Sum{24,26..28,31} (5 alike) : Sum  Inputs=|+-
  Sum25 : Sum  Inputs=|++
  sin ret : Gain  Gain=18
  Out1 : Outport
  Out2 : Outport  Port=2
  wires:
  Gain26/1 -> Sum28/2
  Glucosa basal  4/1 -> Gain22/1, Gain21/1
  D/1 -> Sum24/1
  Gain21/1 -> Gráfica glucosa 4/2  "glucosa basal"
  Integrator11/1 -> sin ret/1, Out2/1, Gain24/1, Product8/1  "G(t)"
  Integrator12/1 -> Product8/2, Gain23/1, Gráfica insulina activa4/1  "X(t)"
  Gain25/1 -> Sum26/1
  Integrator10/1 -> Out1/1, Gráfica insulina 4/1, Sum31/1, Gain26/1  "I(t)"
  Constant5/1 -> Integrator10/2
  Sum31/1 -> Gain25/1
  Sum26/1 -> Integrator12/1
  Gain23/1 -> Sum26/2
  Sum28/1 -> Integrator10/1
  Sum24/1 -> Sum27/1
  Sum25/1 -> Integrator11/1
  Gain24/1 -> Sum24/2
  Insulina basal      4/1 -> Gráfica insulina 4/2
  Sum27/1 -> Sum25/1
  Insulina basal    4/1 -> Sum31/2
  Divide4/1 -> Sum28/1
  Gain22/1 -> Sum25/2
  Product8/1 -> Sum27/2
  Constant4/1 -> Divide4/2
  Constant/1 -> Integrator11/2
  Controlador/1 -> Divide4/1
  sin ret/1 -> Gráfica glucosa 4/1

== matlab function ModelosTFG/Ingesta 75 g2 ==
  data: in input; D output
function D = comida(in)
% Variables de entrada en la funcion
t = in(1) %- 8*60*60; % Ajuste para iniciar a las 8 de la mañana
 
% Parámetros del modelo
Ag = 0.8; % adimensional
Tmaxi = 55*60; % s
Vg = 13.79; % L
Tmaxg = 40*60; % s
t1 = 0;
Dg = 0;
f = 1000/180; % factor de conversión de g a mmol
 
% Comidas (perturbaciones) a lo largo de un día
Dg = 50*f;
% Ecuación
D = (Dg*Ag*(t-t1)*exp(-(t-t1)/Tmaxi))/(Vg*Tmaxg^2);

== matlab function ModelosTFG/Ingesta 75 g3 ==
  data: in input; D output
function D = comida(in)
% Variables de entrada en la funcion
t = in(1) %- 8*60*60; % Ajuste para iniciar a las 8 de la mañana
 
% Parámetros del modelo
Ag = 0.8; % adimensional
Tmaxi = 55*60; % s
Vg = 13.79; % L
Tmaxg = 40*60; % s
t1 = 0;
Dg = 0;
f = 1000/180; % factor de conversión de g a mmol
 
% Comidas (perturbaciones) a lo largo de un día
Dg = 50*f;
% Ecuación
D = (Dg*Ag*(t-t1)*exp(-(t-t1)/Tmaxi))/(Vg*Tmaxg^2);

== matlab function ModelosTFG/Ingesta 75 g4 ==
  data: in input; D output
function D = comida(in)
% Variables de entrada en la funcion
t = in(1) %- 8*60*60; % Ajuste para iniciar a las 8 de la mañana
 
% Parámetros del modelo
Ag = 0.8; % adimensional
Tmaxi = 55*60; % s
Vg = 13.79; % L
Tmaxg = 40*60; % s
t1 = 0;
Dg = 0;
f = 1000/180; % factor de conversión de g a mmol
 
% Comidas (perturbaciones) a lo largo de un día
Dg = 50*f;
% Ecuación
D = (Dg*Ag*(t-t1)*exp(-(t-t1)/Tmaxi))/(Vg*Tmaxg^2);

== matlab function ModelosTFG/Ingesta 75 g9 ==
  data: in input; D output
function D = comida(in)
% Variables de entrada en la funcion
t = in(1) %- 8*60*60; % Ajuste para iniciar a las 8 de la mañana
 
% Parámetros del modelo
Ag = 0.8; % adimensional
Tmaxi = 55*60; % s
Vg = 13.79; % L
Tmaxg = 40*60; % s
t1 = 0;
Dg = 0;
f = 1000/180; % factor de conversión de g a mmol
 
% Comidas (perturbaciones) a lo largo de un día
Dg = 50*f;
% Ecuación
D = (Dg*Ag*(t-t1)*exp(-(t-t1)/Tmaxi))/(Vg*Tmaxg^2);

== matlab function ModelosTFG/Ingesta 75 g10 ==
  data: in input; D output
function D = comida(in)
% Variables de entrada en la funcion
t = in(1) %- 8*60*60; % Ajuste para iniciar a las 8 de la mañana
 
% Parámetros del modelo
Ag = 0.8; % adimensional
Tmaxi = 55*60; % s
Vg = 13.79; % L
Tmaxg = 40*60; % s
t1 = 0;
Dg = 0;
f = 1000/180; % factor de conversión de g a mmol
 
% Comidas (perturbaciones) a lo largo de un día
Dg = 50*f;
 
% Ecuación
D = (Dg*Ag*(t-t1)*exp(-(t-t1)/Tmaxi))/(Vg*Tmaxg^2);

== matlab function ModelosTFG/Ingesta 75 g11 ==
  data: in input; D output
function D = comida(in)
% Variables de entrada en la funcion
t = in(1) %- 8*60*60; % Ajuste para iniciar a las 8 de la mañana
 
% Parámetros del modelo
Ag = 0.8; % adimensional
Tmaxi = 55*60; % s
Vg = 13.79; % L
Tmaxg = 40*60; % s
t1 = 0;
Dg = 0;
f = 1000/180; % factor de conversión de g a mmol
 
% Comidas (perturbaciones) a lo largo de un día
Dg = 50*f;
 
% Ecuación
D = (Dg*Ag*(t-t1)*exp(-(t-t1)/Tmaxi))/(Vg*Tmaxg^2);

== matlab function ModelosTFG/Ingesta 75 g1 ==
  data: in input; D output
function D = comida(in)
% Variables de entrada en la funcion
t = in(1) %- 8*60*60; % Ajuste para iniciar a las 8 de la mañana
 
% Parámetros del modelo
Ag = 0.8; % adimensional
Tmaxi = 55*60; % s
Vg = 13.79; % L
Tmaxg = 40*60; % s
t1 = 0;
Dg = 0;
f = 1000/180; % factor de conversión de g a mmol
 
% Comidas (perturbaciones) a lo largo de un día
%if t >= 0 && t < 180*60 % ingesta de 75 g de HC
   % t1 = 0;
    %Dg = 50*f;
%end
Dg = 50*f;
% Ecuación
D = (Dg*Ag*(t-t1)*exp(-(t-t1)/Tmaxi))/(Vg*Tmaxg^2);
